simulink model "Simulink_deliverable_1"  (R2024b)
settings: Solver=ode4  StartTime=0.0  StopTime=110  FixedStep=1e-3  RelTol=1e-3
settings Model: Creator=20233602  LastModifiedBy=20233602

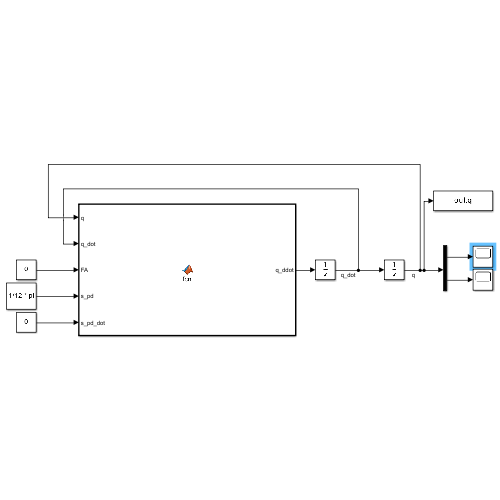
[thumbnail: Simulink's stored preview of the top-level diagram]
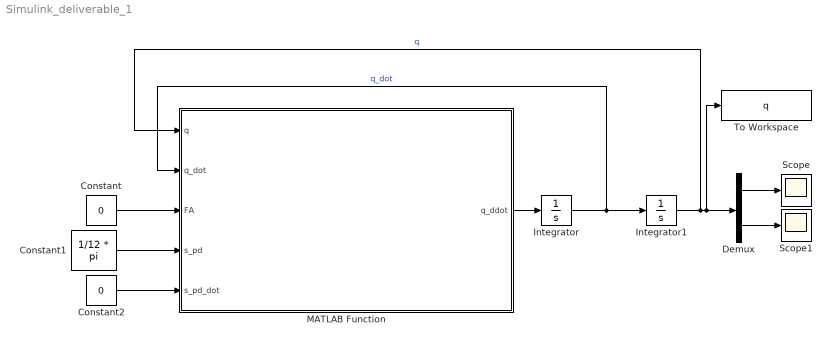
== system Simulink_deliverable_1 ==
  Constant : Constant  Value=0
  Constant1 : Constant  Value=1/12 * pi
  Constant2 : Constant  Value=0
  Demux : Demux  Outputs=2
  Integrator : Integrator  InitialCondition=[0,0]
  Integrator1 : Integrator  InitialCondition=[11.5 , pi/3]
  MATLAB Function : MATLAB Function  TreatAsAtomicUnit=on
  Scope : Scope
  Scope1 : Scope
  To Workspace : ToWorkspace  VariableName=q  SampleTime=-1
  wires:
  Constant/1 -> MATLAB Function/3(FA)
  Constant1/1 -> MATLAB Function/4(s_pd)
  Constant2/1 -> MATLAB Function/5(s_pd_dot)
  MATLAB Function/1(q_ddot) -> Integrator/1
  Integrator/1 -> MATLAB Function/2(q_dot), Integrator1/1  "q_dot"
  Integrator1/1 -> MATLAB Function/1(q), To Workspace/1, Demux/1  "q"
  Demux/2 -> Scope1/1
  Demux/1 -> Scope/1

== matlab function Simulink_deliverable_1/MATLAB Function ==
  data: q input; q_ddot output; q_dot input; FA input; s_pd input; s_pd_dot input
function q_ddot = fcn(q, q_dot, FA, s_pd, s_pd_dot)
%Constants
g = 9.81;
L2 = 10;
m2 = 2000;
m3 = 500;
dW = 2000;
dx = 200;
kx = 7000;
k_theta = 200;
x0 = 11.5;
theta0 = pi/3;

%Generalized constants
x = q(1);
theta = q(2);
x_dot = q_dot(1);
theta_dot = q_dot(2);

%M and F
M = [m2 + m3, L2*m3*sin(s_pd - theta);
    L2*m3*sin(s_pd-theta), L2^2*m3];

F = [-dx*x_dot + FA - kx*(x - x0) + (m2 + m3) *s_pd_dot^2 * x ...
     - g*(m2 + m3) * sin(s_pd) + L2 * m3 * theta_dot^2* cos(s_pd - theta)...
     + L2 * m3 *s_pd_dot * theta_dot * cos(s_pd - theta);
     - dW * theta_dot - k_theta * (theta - theta0) + L2 *g * m3*cos(theta) ...
     - L2*m3*s_pd_dot*x_dot*cos(s_pd-theta)];

q_ddot= transpose(M\F);
